simulink model "MF007_MotVltgSVPWM"  (R2022b)
settings: configuration reference "ASW_Configuration_Set_100ms" (kept outside this file)
values from neighbouring files (symbols this model uses):
  MotCtrlModeEnum : value not decoded    [XPSbW_PublicDataType.sldd]
undefined symbols (not defined in the file or in its folder): CalC_MF007_b_ManMotPwmCtrlEna_UL, CalC_MF007_f32_1D3_UL, CalC_MF007_f32_BrdgVoltFbkFilCoeff_UL, CalC_MF007_f32_ManMotPwmACmd_UL, CalC_MF007_f32_ManMotPwmBCmd_UL, CalC_MF007_f32_ManMotPwmCCmd_UL, CalC_MF007_f32_MotBrdgVltg_V, CalC_MF007_f32_MotCtrlPWMPeriodHiLimit_UL, CalC_MF007_f32_MotCtrlPWMPeriodLowLimit_UL, CalC_MF007_f32_MotPWMTimeDelay_s, CalC_MF007_f32_MotTen_UL, CalC_MF007_f32_MotThreeHundredAndFifty_UL, CalC_MF007_f32_MotZeroAgCounter_UL, CalC_MF007_f32_MotZeroAgone_UL, CalC_MF007_f32_MotZeroAgthree_UL, CalC_MF007_f32_MotZeroAgtwo_UL, CalC_MF007_f32_MoyBrdgVoltLo_V, CalC_MF007_f32_Neg1D2_UL, CalC_MF007_f32_Sqrt3D2_UL, CalC_MF007_f32_ZeroAgCalVolt_V, CalC_XPSbW_b_MotTypSeln_UL, CalC_XPSbW_b_MotZeroCalsEn_UL, Con_XPSbW_b_True_UL, Con_XPSbW_f32_1D100_UL, Con_XPSbW_f32_1D2_UL, Con_XPSbW_f32_Deg2Rad_UL, Con_XPSbW_f32_ES003MotAgArbdMax_deg, Con_XPSbW_f32_ES003MotAgArbdMin_deg, Con_XPSbW_f32_ES004MotVelElecFildMax_radps, Con_XPSbW_f32_ES004MotVelElecFildMin_radps, Con_XPSbW_f32_ES008EPSSupplyVltgMax_V, Con_XPSbW_f32_ES008EPSSupplyVltgMin_V, Con_XPSbW_f32_NegOne_UL, Con_XPSbW_f32_One_UL, Con_XPSbW_f32_Sqrt3_UL, Con_XPSbW_f32_Sqrt3D3_UL, Con_XPSbW_f32_Two_UL, Con_XPSbW_f32_Zero_UL, Con_XPSbW_u8_Four_UL, Con_XPSbW_u8_One_UL, Con_XPSbW_u8_Two_UL, Con_XPSbW_u8_Zero_UL
libraries: XpengCHASbWLib x63, simulink x4
(part 2 of 2)

== stateflow chart MF007_MotVltgSVPWM/MotVltgSVPWMPer1/MotCtrlStatorVltg/Subsystem1/Chart1 ==
  state start
    en:
    Ua=Con_XPSbW_f32_Zero_UL;
    Ub=Con_XPSbW_f32_Zero_UL;
    Uc=Con_XPSbW_f32_Zero_UL;
    Flag_Ok=Con_XPSbW_b_False_UL;
    Pha_Num=Con_XPSbW_u8_Zero_UL;
    MotCalzeroSts=Con_XPSbW_u8_Zero_UL;
  state [Phi_Avg,Err1,Finished1]=Calc_PhiOffset(Phi,Num) [function]
    (default) -> (junction 177)
    (junction 177) -> (junction 178) [order 1] : [Phi<Con_XPSbW_f32_Zero_UL]
    (junction 177) -> (junction 181) [order 2] : %do nothing%
    (junction 178) -> (junction 180) : {Phi=Phi+Con_XPSbW_f32_ThreeSixty_UL;}
    (junction 180) -> (junction 181)
    (junction 181) -> (junction 78)
    (junction 78) -> (junction 79) [order 1] : [Num==Con_XPSbW_u8_One_UL]
    (junction 78) -> (junction 82) [order 2]
    (junction 79) -> (junction 99) : {Phi_Sum=Phi;
        | Err1=Con_XPSbW_b_False_UL;}
    (junction 82) -> (junction 85) [order 1] : [(single(abs(Phi-Phi_Sum/single((Num-Con_XPSbW_u8_One_UL))))>Ten)&&(single(abs(Phi-Phi_Sum/(Num-Con_XPSbW_u8_One_UL)))<ThreeHundredAndFifty)]
    (junction 82) -> (junction 186) [order 2]
    (junction 85) -> (junction 96) : {Err1=Con_XPSbW_b_True_UL;}
    (junction 186) -> (junction 195) [order 1] : [(Phi_Sum/(Num-Con_XPSbW_u8_One_UL)-Phi)>=ThreeHundredAndFifty]
    (junction 186) -> (junction 188) [order 2] : [(Phi-Phi_Sum/(Num-Con_XPSbW_u8_One_UL))>=ThreeHundredAndFifty]
    (junction 195) -> (junction 201) : {Phi_Sum=Phi_Sum-Con_XPSbW_f32_ThreeSixty_UL;}
    (junction 186) -> (junction 191) [order 3] : %do nothing%
    (junction 188) -> (junction 190) : {Phi=Phi-Con_XPSbW_f32_ThreeSixty_UL;}
    (junction 201) -> (junction 191)
    (junction 190) -> (junction 191)
    (junction 191) -> (junction 87) : {Phi_Sum=Phi_Sum+Phi;
        | Err1=Con_XPSbW_b_False_UL;}
    (junction 87) -> (junction 89) [order 1] : [Num==Con_XPSbW_u8_Four_UL]
    (junction 89) -> (junction 93) : {Finished1=Con_XPSbW_b_True_UL;}
    (junction 87) -> (junction 91) [order 2] : {Finished1=Con_XPSbW_b_False_UL;}
    (junction 93) -> (junction 91)
    (junction 96) -> (junction 93)
    (junction 99) -> (junction 96)
    (junction 91) -> (junction 162) : {Phi_Avg=Phi_Sum/Num;}
  state Err
    en:
    Ua=Con_XPSbW_f32_Zero_UL;
    Ub=Con_XPSbW_f32_Zero_UL;
    Uc=Con_XPSbW_f32_Zero_UL;
    Flag_Ok=Con_XPSbW_b_False_UL;
    MotCalzeroSts=Con_XPSbW_u8_One_UL;
  state forward
    state ClockAngle60
      en:
      Ua=InitVolt1;
      Ub=InitVolt1;
      Uc=InitVolt2;
      Pha_Num=Pha_Num+Con_XPSbW_u8_One_UL;
      MotCalzeroSts=Con_XPSbW_u8_Two_UL;
    state ClockAngle180
      en:
      Ua=InitVolt2;
      Ub=InitVolt1;
      Uc=InitVolt1;
      Pha_Num=Pha_Num+Con_XPSbW_u8_One_UL;
      MotCalzeroSts=Con_XPSbW_u8_Three_UL;
    state ClockAngle300
      en:
      Ua=InitVolt1;
      Ub=InitVolt2;
      Uc=InitVolt1;
      Pha_Num=Pha_Num+Con_XPSbW_u8_One_UL;
      MotCalzeroSts=Con_XPSbW_u8_Four_UL;
    state ClockCalc
      en:
      [Phi_Pos,ErrorA,Finished]=Calc_PhiOffset(Phi_Temp,Pha_Num);
      Phi_Out[Pha_Num]=f32_MotAgArbd_deg;
      MotCalzeroSts=Con_XPSbW_u8_Five_UL;
    (default) -> ClockAngle60
    ClockAngle180 -> (junction 133) : [(Pha_Num==Con_XPSbW_u8_Two_UL)...
        | &&after(Counter,tick)]
    ClockCalc -> ClockAngle180 [order 3] : [Pha_Num==Con_XPSbW_u8_One_UL]
    ClockAngle300 -> (junction 135) : [(Pha_Num==Con_XPSbW_u8_Three_UL)...
        | &&after(Counter,tick)]
    ClockCalc -> ClockAngle300 [order 2] : [Pha_Num==Con_XPSbW_u8_Two_UL]
    ClockAngle60 -> (junction 130) : [(Pha_Num==Con_XPSbW_u8_One_UL...
        | ||Pha_Num==Con_XPSbW_u8_Four_UL)...
        | &&after(Counter,tick)]
    ClockCalc -> ClockAngle60 [order 1] : [Pha_Num==Con_XPSbW_u8_Three_UL]
    (junction 130) -> ClockCalc : {Phi_Temp=(f32_MotAgArbd_deg-Agone);}
    (junction 133) -> ClockCalc : {Phi_Temp=(f32_MotAgArbd_deg-Agtwo);}
    (junction 135) -> ClockCalc : {Phi_Temp=(f32_MotAgArbd_deg-Agthree);}
  state backward
    state Angle60
      en:
      Ua=InitVolt1;
      Ub=InitVolt1;
      Uc=InitVolt2;
      Pha_Num=Pha_Num+Con_XPSbW_u8_One_UL;
      MotCalzeroSts=Con_XPSbW_u8_Six_UL;
    state Angle300
      en:
      Ua=InitVolt1;
      Ub=InitVolt2;
      Uc=InitVolt1;
      Pha_Num=Pha_Num+Con_XPSbW_u8_One_UL;
      MotCalzeroSts=Con_XPSbW_u8_Seven_UL;
    state Angle180
      en:
      Ua=InitVolt2;
      Ub=InitVolt1;
      Uc=InitVolt1;
      Pha_Num=Pha_Num+Con_XPSbW_u8_One_UL;
      MotCalzeroSts=Con_XPSbW_u8_Eight_UL;
    state Calc
      en:
      [Phi_Neg,ErrorA,Finished]=Calc_PhiOffset(Phi_Temp,Pha_Num);
      Phi_Out[Pha_Num+Con_XPSbW_u8_Four_UL]=f32_MotAgArbd_deg;
      MotCalzeroSts=Con_XPSbW_u8_Nine_UL;
    (default) -> Angle60
    Angle60 -> (junction 137) : [(Pha_Num==Con_XPSbW_u8_One_UL...
        | ||Pha_Num==Con_XPSbW_u8_Four_UL)...
        | &&after(Counter,tick)]
    Calc -> Angle60 [order 1] : [Pha_Num==Con_XPSbW_u8_Three_UL]
    Angle300 -> (junction 139) : [(Pha_Num==Con_XPSbW_u8_Two_UL)...
        | &&after(Counter,tick)]
    Calc -> Angle300 [order 3] : [Pha_Num==Con_XPSbW_u8_One_UL]
    Angle180 -> (junction 141) : [(Pha_Num==Con_XPSbW_u8_Three_UL)...
        | &&after(Counter,tick)]
    Calc -> Angle180 [order 2] : [Pha_Num==Con_XPSbW_u8_Two_UL]
    (junction 137) -> Calc : {Phi_Temp=(f32_MotAgArbd_deg-Agone);}
    (junction 139) -> Calc : {Phi_Temp=(f32_MotAgArbd_deg-Agthree);}
    (junction 141) -> Calc : {Phi_Temp=(f32_MotAgArbd_deg-Agtwo);}
  state FinalCalC
    (default) -> (junction 47) : {MotCalzeroSts=Con_XPSbW_u8_Nine_UL+Con_XPSbW_u8_One_UL;}
    (junction 47) -> (junction 49) [order 1] : [(single(abs(Phi_Neg-Phi_Pos))>Con_XPSbW_f32_Five_UL)&&(single(abs(Phi_Neg-Phi_Pos))<ThreeHundredAndFifty)]
    (junction 47) -> (junction 204) [order 2]
    (junction 49) -> (junction 128) : {ErrorA=Con_XPSbW_b_True_UL;
        | Phi_Offset=Con_XPSbW_f32_Zero_UL;}
    (junction 204) -> (junction 206) [order 1] : [single(abs(Phi_Neg-Phi_Pos))>=ThreeHundredAndFifty]
    (junction 204) -> (junction 51) [order 2] : {ErrorA=Con_XPSbW_b_False_UL;
        | Phi_Offset=(Phi_Neg+Phi_Pos)/Con_XPSbW_f32_Two_UL;
        | Flag_Ok=Con_XPSbW_b_True_UL;}
    (junction 206) -> (junction 211) : {ErrorA=Con_XPSbW_b_False_UL;
        | Phi_Offset=(Phi_Neg+Phi_Pos-Con_XPSbW_f32_ThreeSixty_UL)/Con_XPSbW_f32_Two_UL;
        | Flag_Ok=Con_XPSbW_b_True_UL;}
    (junction 211) -> (junction 51)
    (junction 128) -> (junction 211)
    (junction 51) -> (junction 52) : {Ua=Con_XPSbW_f32_Zero_UL;
        | Ub=Con_XPSbW_f32_Zero_UL;
        | Uc=Con_XPSbW_f32_Zero_UL;}
    (junction 52) -> (junction 163) [order 1] : [Phi_Offset<Con_XPSbW_f32_Zero_UL]
    (junction 52) -> (junction 165) [order 2] : {Phi_Offset=Phi_Offset;}
    (junction 163) -> (junction 173) : {Phi_Offset=Phi_Offset+Con_XPSbW_f32_ThreeSixty_UL;}
    (junction 173) -> (junction 165)
  (default) -> start
  start -> forward : [after(Con_XPSbW_f32_Thousand_UL,tick)]
  forward -> Err [order 1] : [ErrorA==Con_XPSbW_b_True_UL]
  forward -> backward [order 2] : [Finished==Con_XPSbW_b_True_UL]{Pha_Num=Con_XPSbW_u8_Zero_UL;Finished=Con_XPSbW_b_False_UL;}
  backward -> Err [order 1] : [ErrorA==Con_XPSbW_b_True_UL]
  backward -> FinalCalC [order 2] : [Finished==Con_XPSbW_b_True_UL]
  FinalCalC -> Err : [ErrorA==Con_XPSbW_b_True_UL]
  data: Phi function_input single; Num function_input uint8; Phi_Avg function_output single; Err1 function_output boolean; Finished1 function_output boolean; ErrorA local boolean; Phi_Sum local single; Phi_Neg local single; Phi_Pos local single; Finished local boolean; Phi_Temp local single; Ua output single; Ub output single; Uc output single; f32_MotAgArbd_deg input single; Phi_Offset output single; Flag_Ok output boolean; InitVolt1 input single; Phi_Out output single size=10; InitVolt2 input single; Con_XPSbW_f32_Zero_UL parameter single; Con_XPSbW_b_False_UL parameter boolean; Con_XPSbW_f32_Thousand_UL parameter single; Con_XPSbW_u8_One_UL parameter uint8; Con_XPSbW_u8_Two_UL parameter uint8; Con_XPSbW_u8_Three_UL parameter uint8; Con_XPSbW_u8_Four_UL parameter uint8; Con_XPSbW_b_True_UL parameter boolean; Con_XPSbW_f32_Two_UL parameter single; Con_XPSbW_f32_ThreeSixty_UL parameter single; Con_XPSbW_f32_Five_UL parameter single; Counter input single; Agone input single; Agthree input single; Agtwo input single; Con_XPSbW_u8_Zero_UL parameter uint8; Pha_Num local uint8; Ten input single; MotCalzeroSts output uint8; Con_XPSbW_u8_Six_UL parameter uint8; Con_XPSbW_u8_Seven_UL parameter uint8; Con_XPSbW_u8_Eight_UL parameter uint8; Con_XPSbW_u8_Nine_UL parameter uint8; Con_XPSbW_u8_Five_UL parameter uint8; ThreeHundredAndFifty input single
